simulink model "corners"  (Simulink 7.1)
settings: Solver=ode45  StartTime=0.0  StopTime=10.0  RelTol=1e-3
undefined symbols (not defined in the file or in its folder): gray, Rec, SDTV
libraries: vipsnks x2, vipconversions x1, vipanalysis x1, dspsrcs4 x1
settings Model: Creator=stevenw  LastModifiedBy=stevenw

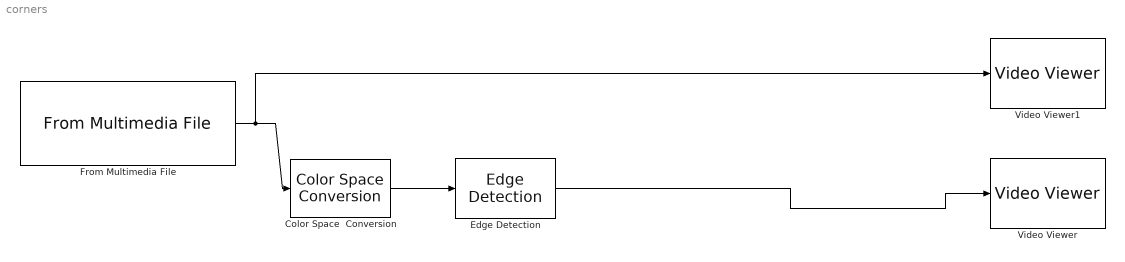
== system corners ==
  Color Space  Conversion : vipconversions/Color Space  Conversion  conversion=Obsolete  conversionActive=R'G'B' to intensity  wp_str=D65  rec=Rec. 601 (SDTV)  sys=1125/60/2:1  imagePorts=One multidimensional signal
  Edge Detection : vipanalysis/Edge Detection  DialogController=vipDDGCreate  DialogControllerArgs=DataTag0  method=Sobel  outputType=Binary image  userDefinedThreshold=off  thresholdSource=Input port  threshold=20  thresholdTuning=4  edgeThinning=off  threshold_canny=[0.25 0.60]  autoPercent=70  sigma=1  prodOutputMode=Binary point scaling  prodOutputWordLength=32  prodOutputFracLength=8  roundingMode=Floor  overflowMode=off
  From Multimedia File : dspsrcs4/From Multimedia File  DialogController=dspDDGCreate  DialogControllerArgs=DataTag1  inputFilename=trafficlanes.avi  loop=on  numPlays=inf  outputStreams=Video only  videoDataType=single  audioDataType=int16  inheritSampleTime=on  userDefinedSampleTime=1/30  noAudioOutput=off  isIntensityVideo=off  colorVideoFormat=One multidimensional signal  outputEOF=off  dataOrg=Column-major
  Video Viewer : vipsnks/Video Viewer  DialogController=vipDDGCreate  DialogControllerArgs=DataTag2  inputType=Obsolete7b  imagePorts=One multidimensional signal  useColorMap=off  colormapValue=gray(256)  specRange=off  minInputVal=0  maxInputVal=255  FigPos=[780 473 360 240]  AxisZoom=on  trueSizedOnce=on
  Video Viewer1 : vipsnks/Video Viewer  DialogController=vipDDGCreate  DialogControllerArgs=DataTag3  inputType=Obsolete7b  imagePorts=One multidimensional signal  useColorMap=off  colormapValue=gray(256)  specRange=off  minInputVal=0  maxInputVal=255  FigPos=[780 473 360 240]  AxisZoom=on  trueSizedOnce=on
  wires:
  From Multimedia File/1 -> Video Viewer1/1, Color Space  Conversion/1
  Edge Detection/1 -> Video Viewer/1
  Color Space  Conversion/1 -> Edge Detection/1
